simulink model "Que2"  (R2023b)
settings: Solver=VariableStepAuto  StartTime=0.0  StopTime=50  RelTol=1e-3
settings Model: Creator=ali14  LastModifiedBy=setak
settings OptimizationCC: ReuseModelBlockBuffer=off

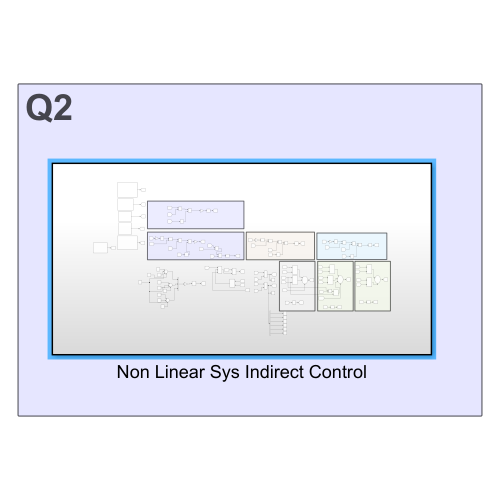
[thumbnail: Simulink's stored preview of the top-level diagram]
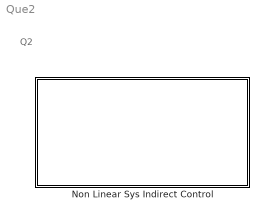
== system Que2 ==
  note: Q2
  Non Linear Sys Indirect Control : Subsystem

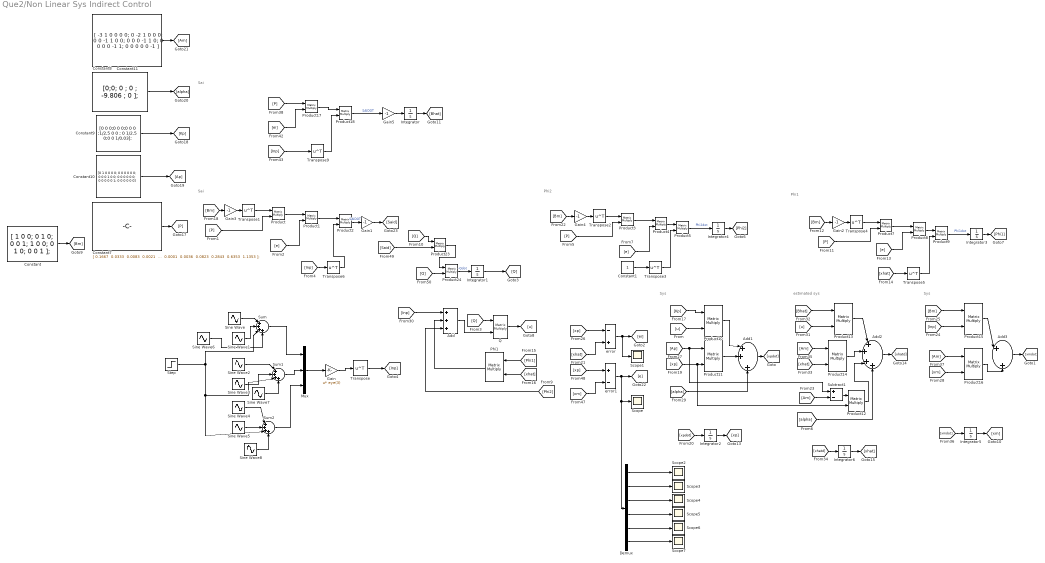
== system Que2/Non Linear Sys Indirect Control ==
  note: Phi1
  note: Sys
  note: Sai
  note: Sys
  note: Sai
  note: Phi2
  note: estimated sys
  Add : Sum  Inputs=+++
  Add1 : Sum  Inputs=|++|+
  Add2 : Sum  Inputs=|+|+|+|+
  Add3 : Sum  Inputs=|+|+
  Constant : Constant  Value=|
      | [ 1 0 0;
      |            0 1 0;
      |            0 0 1;
      |            1 0 0;
      |            0 1 0;
      |            0 0 1 ];
  Constant1 : Constant
  Constant10 : Constant  Value=|
      | [0 1 0 0 0 0;      0 0 0 0 0 0;
      |       0 0 0 1 0 0;      0 0 0 0 0 0;
      |       0 0 0 0 0 1;      0 0 0 0 0 0]
  Constant11 : Constant  Value=|
      | [ -3  1  0  0  0  0;
      |             0 -2  1  0  0  0;
      |             0  0 -1  1  0  0;
      |             0  0  0 -1  1  0;
      |             0  0  0  0 -1  1;
      |             0  0  0  0  0 -1 ]
  Constant7 : Constant  Value=|
      | [ 0.1667  0.0333  0.0083  0.0021  0.0005  0.0001;
      |           0.0333  0.2667  0.0917  0.0312  0.0106  0.0036;
      |           0.0083  0.0917  0.5917  0.3115  0.1610  0.0823;
      |           0.0021  0.0312  0.3115  0.8115  0.4862  0.2843;
      |           0.0005  0.0106  0.1610  0.4862  0.9862  0.6353;
      |           0.0001  0.0036  0.0823  0.2843  0.6353  1.1353 ];
  Constant8 : Constant  Value=|
      | [0;0;      0 ;
      |       0 ;  -9.806 ;      0 ];
  Constant9 : Constant  Value="[0 0 0;0 0 0;0 0 0 ;1/2.5 0 0  ; 0 1/2.5  0;0 0 1/0.03];"
  Demux : Demux  Outputs=6
  Gain : Gain  Gain=eye(3)  Multiplication=Matrix(u*K)
  Gain{1..5} (5 alike) : Gain  Gain=-1
  Integrator{,3..5} (4 alike) : Integrator
  Integrator1 : Integrator  InitialCondition=[0 0 0; 0 0 0; 0 0 0]  IgnoreLimit=on
  Integrator2 : Integrator  InitialCondition=[0 ;0; 0;0;0;0]
  Integrator6 : Integrator  InitialCondition=[0; 0; 0;0;0;0]
  Mux : Mux  Inputs=3
  Phi1 : Product  Multiplication=Matrix(*)
  Product{,1..5,7..18,23..24} (20 alike) : Product  Multiplication=Matrix(*)
  Q : Product  Multiplication=Matrix(*)
  Scope{,1..7} (8 alike) : Scope
  Sine Wave : Sin  SampleTime=0
  Sine Wave1 : Sin  Amplitude=3  Frequency=1.5  SampleTime=0
  Sine Wave2 : Sin  Amplitude=2  Frequency=2  SampleTime=0
  Sine Wave3 : Sin  Amplitude=3  Frequency=2.5  SampleTime=0
  Sine Wave4 : Sin  Amplitude=3  Frequency=3  SampleTime=0
  Sine Wave5 : Sin  Amplitude=4  Frequency=3.5  SampleTime=0
  Sine Wave6 : Sin  Amplitude=2  Frequency=4  SampleTime=0
  Sine Wave7 : Sin  Amplitude=3  Frequency=9  SampleTime=0
  Sine Wave8 : Sin  Amplitude=3  Frequency=4  SampleTime=0
  Step : Step  Before=2  After=3  SampleTime=0
  Subtract1 : Sum  Inputs=+-
  Sum : Sum  Inputs=|++++
  Sum1 : Sum  Inputs=|++++
  Sum2 : Sum  Inputs=|++++
  Transpose{,1..6,9} (8 alike) : Math  Operator=transpose
  error : Sum  Inputs=-+
  error1 : Sum  Inputs=+-
  wires:
  [Q] -> Product24/2
  [xp] -> error1/1
  Product23/1 -> Product24/1
  [ei] -> Product17/2
  Sine Wave4/1 -> Sum2/1
  [Am] -> Subtract1/2
  [alpha] -> Add2/4
  [Said] -> Product23/2
  Constant/1 -> [Bm]
  [Ap] -> Subtract1/1, Product11/1
  [P] -> Product7/2
  Gain1/1 -> [Said]
  [e] -> Product8/2
  [Am] -> Product14/1
  Gain5/1 -> Integrator/1
  [xm] -> error1/2
  [Inp] -> Transpose6/1
  Transpose9/1 -> Product18/2
  [e] -> Product1/2
  Add2/1 -> [xhatd]
  Product24/1 -> Integrator1/1  "-Qdot"
  Sine Wave2/1 -> Sum1/1
  Product17/1 -> Product18/1
  Integrator2/1 -> [xp]
  [xp] -> Product12/2, Product11/2
  Add1/1 -> [xpdot]
  [alpha] -> Add1/3
  Integrator4/1 -> [Phi2]
  Product13/1 -> Add2/1
  Product3/1 -> Product4/1
  Constant10/1 -> [Ap]
  Integrator1/1 -> [Q]
  Step/1 -> Sum2/3, Sum1/3, Sum/3
  Sine Wave3/1 -> Sum1/2
  [P] -> Product17/1
  [xm] -> Product16/2
  Integrator5/1 -> [xm]
  Constant9/1 -> [Kp]
  [Inp] -> Transpose9/1
  Product1/1 -> Product2/1
  [Kp] -> Product10/1
  Product12/1 -> Add2/3
  [Inp] -> Product15/2
  Product15/1 -> Add3/1
  [Bm] -> Gain4/1
  [Inp] -> Add/1
  Add3/1 -> [xmdot]
  [Bm] -> Product15/1
  Subtract1/1 -> Product12/1
  Integrator3/1 -> [Phi1]
  Transpose/1 -> [Inp]
  [Bhat] -> Product13/1
  Mux/1 -> Gain/1
  Product11/1 -> Add1/2
  Product8/1 -> Product9/1
  [xhatd] -> Integrator6/1
  Integrator/1 -> [Bhat]
  Sine Wave/1 -> Sum/1
  Transpose6/1 -> Product2/2
  [Phi1] -> Phi1/1
  Sum2/1 -> Mux/3
  [Phi2] -> Add/3
  Sum/1 -> Mux/1
  Product5/1 -> Integrator4/1  "Phi2dot"
  Sum1/1 -> Mux/2
  Product16/1 -> Add3/2
  Sine Wave1/1 -> Sum/2
  [Bm] -> Gain2/1
  Product14/1 -> Add2/2
  [xhat] -> Phi1/2
  Phi1/1 -> Add/2
  [P] -> Product3/2
  Transpose5/1 -> Product9/2
  Product/1 -> Product1/1
  [P] -> Product/2
  error/1 -> Scope1/1, [ei]
  [xhat] -> Product14/2
  Gain4/1 -> Transpose2/1
  [xp] -> error/1
  Transpose2/1 -> Product3/1
  Product2/1 -> Gain1/1  "SAIDOT"
  [u] -> Product10/2
  Product9/1 -> Integrator3/1  "Phi1dot"
  [xpdot] -> Integrator2/1
  [Q] -> Q/1
  [Bm] -> Gain3/1
  Gain/1 -> Transpose/1
  [xmdot] -> Integrator5/1
  Transpose1/1 -> Product/1
  Product10/1 -> Add1/1
  [Am] -> Product16/1
  [e] -> Product4/2
  Sine Wave5/1 -> Sum2/2
  Product18/1 -> Gain5/1  "SAIDOT"
  Constant7/1 -> [P]
  Add/1 -> Q/2
  [xhat] -> Transpose5/1
  [xhat] -> error/2
  Gain2/1 -> Transpose4/1
  Product4/1 -> Product5/1
  Q/1 -> [u]
  Transpose4/1 -> Product7/1
  Transpose3/1 -> Product5/2
  Constant11/1 -> [Am]
  Product7/1 -> Product8/1
  Constant1/1 -> Transpose3/1
  [u] -> Product13/2
  Constant8/1 -> [alpha]
  Integrator6/1 -> [xhat]
  Gain3/1 -> Transpose1/1
  [Q] -> Product23/1
  Demux/6 -> Scope7/1
  error1/1 -> Demux/1, Scope/1, [e]
  Demux/5 -> Scope6/1
  Demux/1 -> Scope2/1
  Demux/2 -> Scope3/1
  Demux/3 -> Scope4/1
  Demux/4 -> Scope5/1
  Sine Wave6/1 -> Sum/4
  Sine Wave7/1 -> Sum1/4
  Sine Wave8/1 -> Sum2/4
